simulink model "lab01"  (R2025a)
settings: Solver=VariableStepAuto  StartTime=0.0  StopTime=10.0  RelTol=1e-3
settings Model: Creator=grigorijtomczuk  LastModifiedBy=grigorijtomczuk

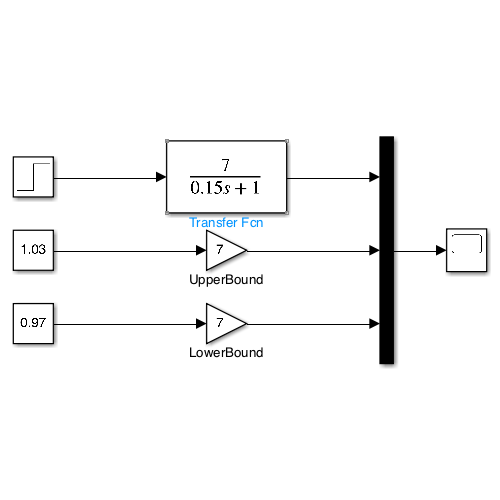
[thumbnail: Simulink's stored preview of the top-level diagram]
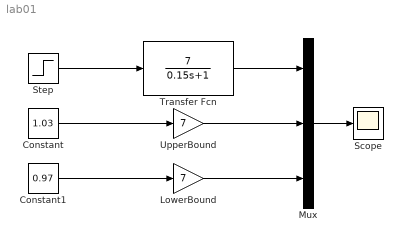
== system lab01 ==
  Constant : Constant  Value=1.03
  Constant1 : Constant  Value=0.97
  LowerBound : Gain  Gain=7
  Mux : Mux  Inputs=3
  Scope : Scope
      settings: ActiveDisplayYMinimum=-0.90124999999999977  ActiveDisplayYMaximum=8.11125
  Step : Step  SampleTime=0
  Transfer Fcn : TransferFcn  Numerator=[7]  Denominator=[0.15 1]
  UpperBound : Gain  Gain=7
  wires:
  Constant/1 -> UpperBound/1
  Constant1/1 -> LowerBound/1
  Step/1 -> Transfer Fcn/1
  Transfer Fcn/1 -> Mux/1
  UpperBound/1 -> Mux/2
  LowerBound/1 -> Mux/3
  Mux/1 -> Scope/1
